simulink model "classicMRAC"  (R2022b)
settings: Solver=VariableStepAuto  StartTime=0.0  StopTime=10.0  RelTol=1e-3
values from neighbouring files (symbols this model uses):
  a_plant = -10    [runClassicMRAC.m]
  alpha0 = 0    [Run_Both_Model.m]    (also in Run_Deadzone.m; Run_ScalarModel.m; Slicing.m; UniCenterMRAC.m)
  ar = -20    [Run_Both_Model.m]    (also in Run_Deadzone.m; Run_Project1i_haoran9.m; Run_ScalarModel.m; Slicing.m)
  b_plant = +10    (= 10)    [runClassicMRAC.m]
  beta0 = 0    [Run_Both_Model.m]    (also in Run_Deadzone.m; Run_ScalarModel.m; Slicing.m; UniCenterMRAC.m)
  br = 20    [Run_Both_Model.m]    (also in Run_Deadzone.m; Run_Project1i_haoran9.m; Run_ScalarModel.m; Slicing.m)
  ga = 10    [Run_Both_Model.m]    (also in Run_Deadzone.m; Run_ScalarModel.m; Slicing.m; UniCenterMRAC.m = 0)
  gb = 10    [Run_Both_Model.m]    (also in Run_Deadzone.m; Run_ScalarModel.m; Slicing.m; UniCenterMRAC.m = 0)
  sigma = 0.1    [Run_Both_Model.m]    (also in Run_Deadzone.m; Run_Project1i_haoran9.m; Run_ScalarModel.m; Slicing.m)
  x0 = 0    [Run_Both_Model.m]    (also in Run_Deadzone.m; Run_Project1i_haoran9.m = 1; Run_ScalarModel.m; Slicing.m = 5)
  xr0 = 0    [Run_Both_Model.m]    (also in Run_Deadzone.m; Run_Project1i_haoran9.m; Run_ScalarModel.m; Slicing.m)
libraries: simulink x2
settings Model: Creator=Nathan  LastModifiedBy=Nathan

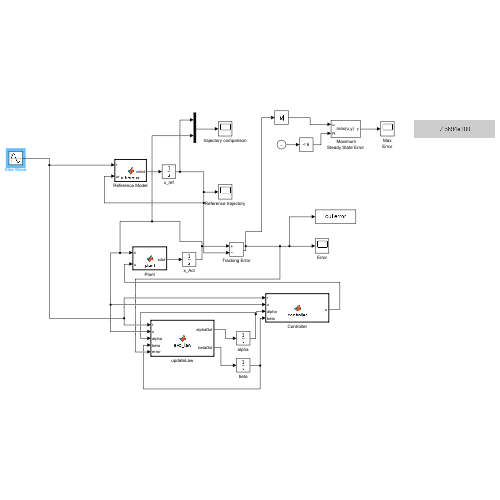
[thumbnail: Simulink's stored preview of the top-level diagram]
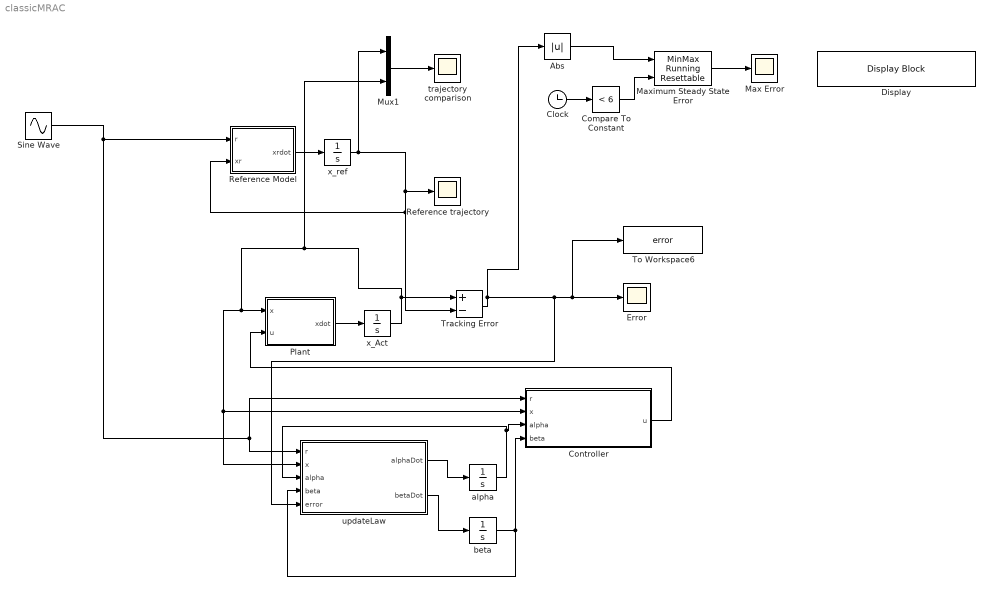
== system classicMRAC ==
  " Maximum Steady State Error" : simulink/Math Operations/MinMax Running Resettable  Function=max  vinit=0.0
  Abs : Abs  SaturateOnIntegerOverflow=off
  Clock : Clock
  Compare To Constant : simulink/Logic and Bit Operations/Compare To Constant  relop=<  const=6  OutDataTypeStr=boolean
  Controller : MATLAB Function  TreatAsAtomicUnit=on
  Display : DisplayBlock  LabelPosition=Hide  Format=shortE  Transparency=1
  Error : Scope
  Max Error : Scope
  Mux1 : Mux  Inputs=2
  Plant : MATLAB Function  TreatAsAtomicUnit=on
  Reference Model : MATLAB Function  TreatAsAtomicUnit=on
  Reference trajectory : Scope
  Sine Wave : Sin  Amplitude=10  Frequency=2  SampleTime=0
  To Workspace6 : ToWorkspace  VariableName=error  SaveFormat=Timeseries  SampleTime=-1
  Tracking Error : Sum  Inputs=+-
  alpha : Integrator  InitialCondition=alpha0
  beta : Integrator  InitialCondition=beta0
  trajectory comparison : Scope
  updateLaw : MATLAB Function  TreatAsAtomicUnit=on
  x_Act : Integrator  InitialCondition=x0
  x_ref : Integrator  InitialCondition=xr0
  wires:
  x_Act/1 -> Mux1/2, updateLaw/2(x), Controller/2(x), Plant/1(x), Tracking Error/1
  Abs/1 -> " Maximum Steady State Error"/1
  updateLaw/2(betaDot) -> beta/1
  Compare To Constant/1 -> " Maximum Steady State Error"/2
  Plant/1(xdot) -> x_Act/1
  " Maximum Steady State Error"/1 -> Max Error/1
  Controller/1(u) -> Plant/2(u)
  updateLaw/1(alphaDot) -> alpha/1
  Tracking Error/1 -> Abs/1, updateLaw/5(error), Error/1, To Workspace6/1
  Mux1/1 -> trajectory comparison/1
  Sine Wave/1 -> Reference Model/1(r), updateLaw/1(r), Controller/1(r)
  Reference Model/1(xrdot) -> x_ref/1
  x_ref/1 -> Reference trajectory/1, Tracking Error/2, Reference Model/2(xr), Mux1/1
  Clock/1 -> Compare To Constant/1
  beta/1 -> Controller/4(beta), updateLaw/4(beta)
  alpha/1 -> updateLaw/3(alpha), Controller/3(alpha)

== matlab function classicMRAC/Reference Model ==
  data: r input; xr input; xrdot output; ar parameter; br parameter
function xrdot = reference(r,xr,ar, br)

xrdot = ar*xr+br*r;

== matlab function classicMRAC/Plant ==
  data: x input; u input; xdot output; a_plant parameter; b_plant parameter
function xdot = plant(x,u,a_plant, b_plant)
f = @(x) -x^3+10*tanh(x);
xdot = a_plant*x+b_plant*(u+f(x));

== matlab function classicMRAC/updateLaw ==
  data: ga parameter; alphaDot output size=1; betaDot output size=1; gb parameter; sigma parameter; r input; x input; alpha input; beta input; error input
function [alphaDot,betaDot]= evo_law(ga, gb,  sigma, r, x, alpha, beta, error)
%% Classic Case
alphaDot=-ga*x*error-sigma*alpha;
betaDot=-gb*r*error-sigma*beta;

== matlab function classicMRAC/Controller ==
  data: r input; u output size=1; x input; alpha input; beta input
function u = controller(r, x,alpha,beta)

% Classic
u = alpha*x+beta*r;
